simulink model "PMSG_Quantum_Main"  (R2024a)
settings: Solver=ode45  StartTime=0.0  StopTime=6.0  RelTol=1e-3
settings Model: Creator=saranboddu  LastModifiedBy=saranboddu

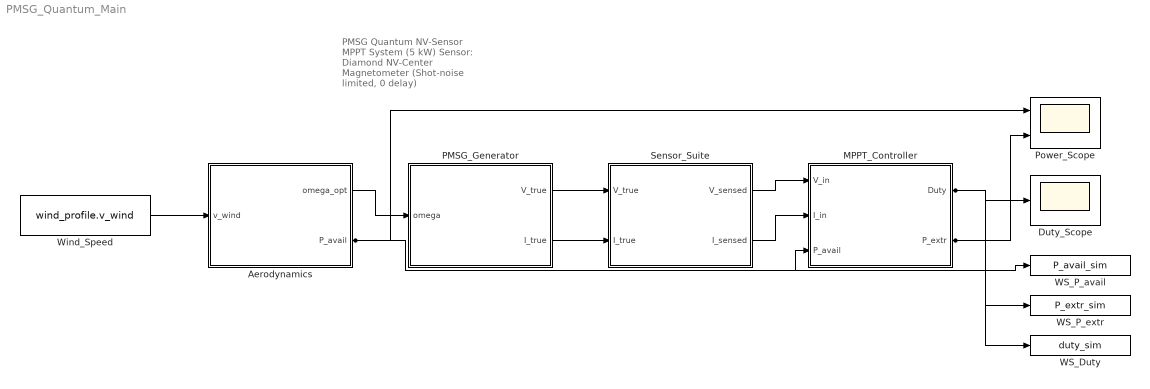
== system PMSG_Quantum_Main ==
  note: PMSG Quantum NV-Sensor MPPT System (5 kW)
      | Sensor: Diamond NV-Center Magnetometer (Shot-noise limited, 0 delay)
  Aerodynamics : Subsystem
  Duty_Scope : Scope
  MPPT_Controller : Subsystem
  PMSG_Generator : Subsystem
  Power_Scope : Scope  NumInputPorts=2
  Sensor_Suite : Subsystem
  WS_Duty : ToWorkspace  VariableName=duty_sim  SampleTime=-1
  WS_P_avail : ToWorkspace  VariableName=P_avail_sim  SampleTime=-1
  WS_P_extr : ToWorkspace  VariableName=P_extr_sim  SampleTime=-1
  Wind_Speed : FromWorkspace  VariableName=wind_profile.v_wind  SampleTime=-1
  wires:
  Wind_Speed/1 -> Aerodynamics/1(v_wind)
  Aerodynamics/1(omega_opt) -> PMSG_Generator/1(omega)
  PMSG_Generator/1(V_true) -> Sensor_Suite/1(V_true)
  PMSG_Generator/2(I_true) -> Sensor_Suite/2(I_true)
  Sensor_Suite/1(V_sensed) -> MPPT_Controller/1(V_in)
  Sensor_Suite/2(I_sensed) -> MPPT_Controller/2(I_in)
  Aerodynamics/2(P_avail) -> MPPT_Controller/3(P_avail), Power_Scope/1, WS_P_avail/1
  MPPT_Controller/1(Duty) -> Duty_Scope/1, WS_Duty/1
  MPPT_Controller/2(P_extr) -> Power_Scope/2, WS_P_extr/1

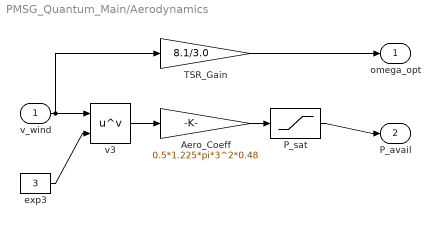
== system PMSG_Quantum_Main/Aerodynamics ==
  v_wind : Inport
  Aero_Coeff : Gain  Gain=0.5*1.225*pi*3^2*0.48
  P_sat : Saturate  UpperLimit=5000  LowerLimit=0
  TSR_Gain : Gain  Gain=8.1/3.0
  exp3 : Constant  Value=3
  v3 : Math  Operator=pow
  omega_opt : Outport
  P_avail : Outport  Port=2
  wires:
  ? -> ?
  v_wind/1 -> v3/1, TSR_Gain/1
  exp3/1 -> v3/2
  v3/1 -> Aero_Coeff/1
  Aero_Coeff/1 -> P_sat/1
  P_sat/1 -> P_avail/1
  TSR_Gain/1 -> omega_opt/1

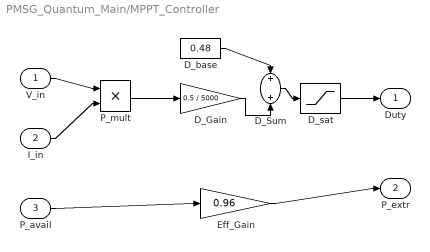
== system PMSG_Quantum_Main/MPPT_Controller ==
  V_in : Inport
  I_in : Inport  Port=2
  P_avail : Inport  Port=3
  D_Gain : Gain  Gain=0.5 / 5000
  D_Sum : Sum
  D_base : Constant  Value=0.48
  D_sat : Saturate  UpperLimit=0.9  LowerLimit=0.1
  Eff_Gain : Gain  Gain=0.96
  P_mult : Product
  Duty : Outport
  P_extr : Outport  Port=2
  wires:
  ? -> ?
  V_in/1 -> P_mult/1
  I_in/1 -> P_mult/2
  P_mult/1 -> D_Gain/1
  D_base/1 -> D_Sum/1
  D_Gain/1 -> D_Sum/2
  D_Sum/1 -> D_sat/1
  D_sat/1 -> Duty/1
  P_avail/1 -> Eff_Gain/1
  Eff_Gain/1 -> P_extr/1

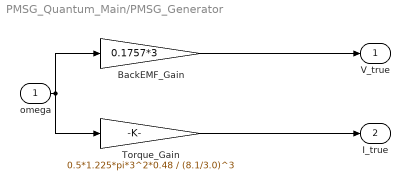
== system PMSG_Quantum_Main/PMSG_Generator ==
  omega : Inport
  BackEMF_Gain : Gain  Gain=0.1757*3
  Torque_Gain : Gain  Gain=0.5*1.225*pi*3^2*0.48 / (8.1/3.0)^3
  V_true : Outport
  I_true : Outport  Port=2
  wires:
  ? -> ?
  omega/1 -> BackEMF_Gain/1, Torque_Gain/1
  BackEMF_Gain/1 -> V_true/1
  Torque_Gain/1 -> I_true/1

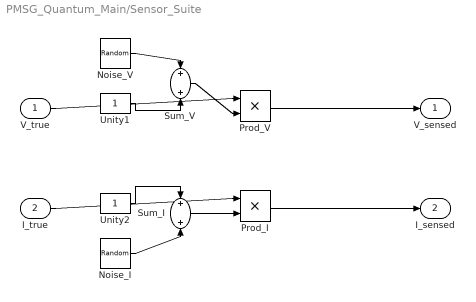
== system PMSG_Quantum_Main/Sensor_Suite ==
  V_true : Inport
  I_true : Inport  Port=2
  Noise_I : RandomNumber  Variance=1e-6  SampleTime=1e-4
  Noise_V : RandomNumber  Variance=1e-6  SampleTime=1e-4
  Prod_I : Product
  Prod_V : Product
  Sum_I : Sum
  Sum_V : Sum
  Unity1 : Constant
  Unity2 : Constant
  V_sensed : Outport
  I_sensed : Outport  Port=2
  wires:
  ? -> ?
  Noise_V/1 -> Sum_V/1
  Unity1/1 -> Sum_V/2
  V_true/1 -> Prod_V/1
  Sum_V/1 -> Prod_V/2
  Prod_V/1 -> V_sensed/1
  Noise_I/1 -> Sum_I/2
  Unity2/1 -> Sum_I/1
  I_true/1 -> Prod_I/1
  Sum_I/1 -> Prod_I/2
  Prod_I/1 -> I_sensed/1
